simulink model "lpa1"  (R2024a)
settings: Solver=FixedStepDiscrete  StartTime=0.0  StopTime=6  FixedStep=0.01  RelTol=1e-3
undefined symbols (not defined in the file): DiscIntNeverNeededParam
settings Model: SILPILSimulationModeModelRef=accelerator  Creator=Anas  LastModifiedBy=Anas
settings OptimizationCC: DefaultParameterBehavior=Inlined  EnhancedBackFolding=on  PassReuseOutputArgsAs=Individual arguments  ZeroExternalMemoryAtStartup=off  ZeroInternalMemoryAtStartup=off  OptimizeBlockOrder=speed  DifferentSizesBufferReuse=on  OptimizationCustomize=off  EfficientTunableParamExpr=on
settings DebuggingCC: ParameterTunabilityLossMsg=error
settings SFSimCC: MATLABDynamicMemAlloc=off
settings RTWCC: Description=Embedded Coder  SystemTargetFile=ert.tlc  TemplateMakefile=ert_default_tmf  Toolchain=MinGW64 | gmake (64-bit Windows)
settings CodeAppCC: ForceParamTrailComments=on  IgnoreCustomStorageClasses=off  OperatorAnnotations=on  SimulinkDataObjDesc=on  SFDataObjDesc=on  InsertBlockDesc=on
settings ERTTargetCC: TargetLangStandard=C99 (ISO)  GenerateSampleERTMain=on  InlinedParameterPlacement=NonHierarchical  ERTCustomFileTemplate=example_file_process.tlc
settings ConfigComp: CovEnable=on  RecordCoverage=on  CovMetricSettings=dcmwe  CovModelRefEnable=on  DVTestSuiteOptimization=Auto  DVDetectOutOfBounds=on  DVModelReferenceHarness=on  DVHarnessSource=Signal Editor

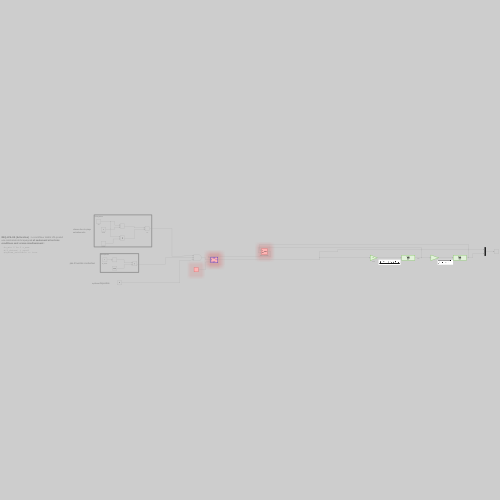
[thumbnail: Simulink's stored preview of the top-level diagram]
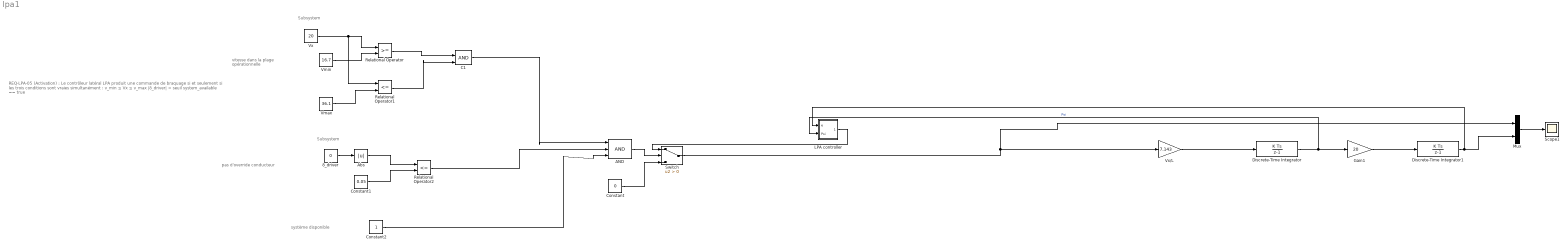
== system lpa1 ==
  note: REQ-LPA-05 (Activation) : Le contrôleur latéral LPA produit une commande de braquage si et seulement si les trois conditions sont vraies simultanément :
      | v_min ≤ Vx ≤ v_max
      | |δ_driver| < seuil
      | system_available == true
  note: Subsystem
  note: Subsystem
  note: vitesse dans la plage opérationnelle
  note: pas d'override conducteur
  note: système disponible
  AND : Logic  Inputs=3  IconShape=distinctive  AllPortsSameDT=off  OutDataTypeStr=boolean
  Abs : Abs  SaturateOnIntegerOverflow=off
  C1 : Logic  IconShape=distinctive  AllPortsSameDT=off  OutDataTypeStr=boolean
  Constant : Constant  Value=0
  Constant1 : Constant  Value=0.05
  Constant2 : Constant
  Discrete-Time Integrator : DiscreteIntegrator  SampleTime=0.01  ICPrevOutput=DiscIntNeverNeededParam  ICPrevScaledInput=DiscIntNeverNeededParam
  Discrete-Time Integrator1 : DiscreteIntegrator  InitialCondition=0.5  SampleTime=0.01  ICPrevOutput=DiscIntNeverNeededParam  ICPrevScaledInput=DiscIntNeverNeededParam
  Gain1 : Gain  Gain=20
  LPA controller : Subsystem  TreatAsAtomicUnit=on  SystemSampleTime=0.01
  Mux : Mux  Inputs=2
  Relational Operator : RelationalOperator  OutDataTypeStr=boolean  RndMeth=Simplest  InputSameDT=off
  Relational Operator1 : RelationalOperator  Operator=<=  OutDataTypeStr=boolean  RndMeth=Simplest  InputSameDT=off
  Relational Operator2 : RelationalOperator  Operator=<=  OutDataTypeStr=boolean  RndMeth=Simplest  InputSameDT=off
  Scope1 : Scope
  Switch : Switch  Criteria=u2 > Threshold  SaturateOnIntegerOverflow=off  InputSameDT=off
  Vmax : Constant  Value=36.1
  Vmin : Constant  Value=16.7
  Vx : Constant  Value=20
  Vx/L : Gain  Gain=7.143
  δ_driver : Constant  Value=0
  wires:
  Vx/L/1 -> Discrete-Time Integrator/1
  Discrete-Time Integrator/1 -> LPA controller/2(Psi), Gain1/1  "Psi"
  Gain1/1 -> Discrete-Time Integrator1/1
  Discrete-Time Integrator1/1 -> LPA controller/1(e), Mux/2
  Mux/1 -> Scope1/1
  Switch/1 -> Mux/1, Vx/L/1
  AND/1 -> Switch/2
  Constant/1 -> Switch/3
  C1/1 -> AND/1
  Vmin/1 -> Relational Operator/2
  Relational Operator/1 -> C1/1
  Vmax/1 -> Relational Operator1/2
  Relational Operator1/1 -> C1/2
  Vx/1 -> Relational Operator1/1, Relational Operator/1
  Relational Operator2/1 -> AND/2
  δ_driver/1 -> Abs/1
  Constant1/1 -> Relational Operator2/2
  Abs/1 -> Relational Operator2/1
  Constant2/1 -> AND/3
  LPA controller/1(delta) -> Switch/1

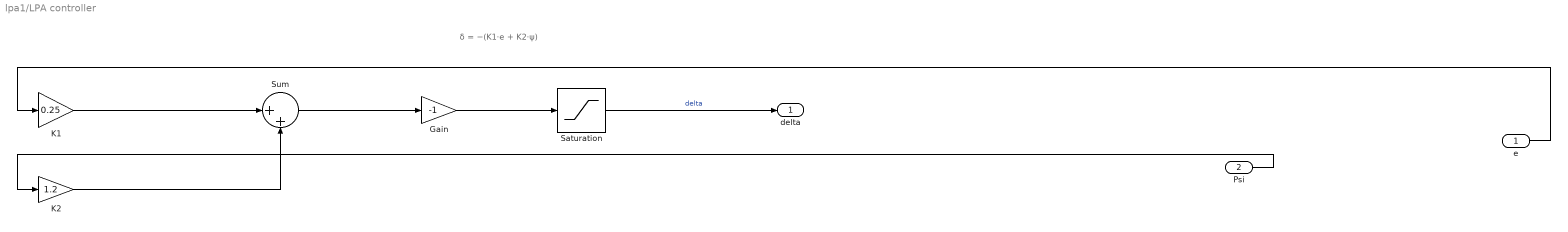
== system lpa1/LPA controller ==
  note: δ = −(K1·e + K2·ψ)
  e : Inport
  Psi : Inport  Port=2
  Gain : Gain  Gain=-1
  K1 : Gain  Gain=0.25
  K2 : Gain  Gain=1.2
  Saturation : Saturate
  Sum : Sum  Inputs=|++
  delta : Outport
  wires:
  Sum/1 -> Gain/1
  K1/1 -> Sum/1
  Gain/1 -> Saturation/1
  e/1 -> K1/1
  K2/1 -> Sum/2
  Saturation/1 -> delta/1  "delta"
  Psi/1 -> K2/1
